simulink model "modelo_sistema"  (R2018b)
settings: Solver=ode3  StartTime=0.0  StopTime=10.0  FixedStep=1e-3  RelTol=1e-3
undefined symbols (not defined in the file): B, F, m
libraries: simulink x1
settings Model: Creator=yasminnunes  LastModifiedBy=yasminnunes

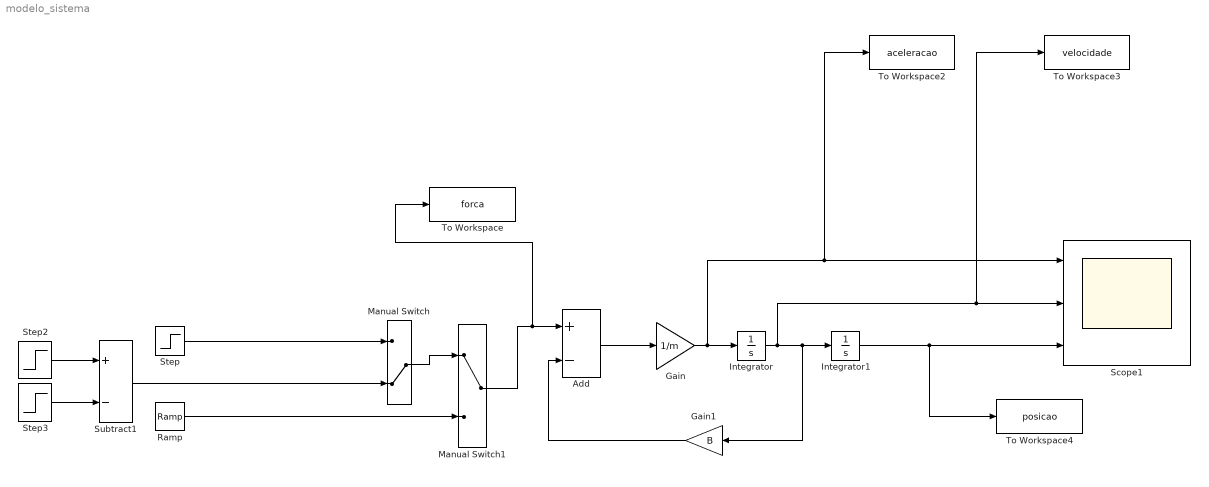
== system modelo_sistema ==
  Add : Sum  Inputs=+-
  Gain : Gain  Gain=1/m
  Gain1 : Gain  Gain=B
  Integrator : Integrator
  Integrator1 : Integrator
  Manual Switch : ManualSwitch  CurrentSetting=0
  Manual Switch1 : ManualSwitch
  Ramp : simulink/Sources/Ramp  slope=F  start=0  InitialOutput=0
  Scope1 : Scope  NumInputPorts=3
  Step : Step  After=F  SampleTime=0
  Step2 : Step  After=F  SampleTime=0
  Step3 : Step  Time=1.1  After=10  SampleTime=0
  Subtract1 : Sum  Inputs=+-
  To Workspace : ToWorkspace  VariableName=forca  SampleTime=-1
  To Workspace2 : ToWorkspace  VariableName=aceleracao  SampleTime=-1
  To Workspace3 : ToWorkspace  VariableName=velocidade  SampleTime=-1
  To Workspace4 : ToWorkspace  VariableName=posicao  SampleTime=-1
  wires:
  Step/1 -> Manual Switch/1
  Add/1 -> Gain/1
  Gain1/1 -> Add/2
  Manual Switch/1 -> Manual Switch1/1
  Ramp/1 -> Manual Switch1/2
  Subtract1/1 -> Manual Switch/2
  Step3/1 -> Subtract1/2
  Step2/1 -> Subtract1/1
  Gain/1 -> Scope1/1, To Workspace2/1, Integrator/1
  Integrator/1 -> To Workspace3/1, Scope1/2, Gain1/1, Integrator1/1
  Integrator1/1 -> To Workspace4/1, Scope1/3
  Manual Switch1/1 -> To Workspace/1, Add/1
